simulink model "video_QPSK"  (R2024b)
settings: Solver=VariableStepAuto  StartTime=0.0  StopTime=10.0  RelTol=1e-3
values from neighbouring files (symbols this model uses):
  frame_rate = video.FrameRate    [vid.m]
undefined symbols (not defined in the file or in its folder): doppler, j
libraries: dspxfrm3 x3, commchan3 x2, commdigbbndpm3 x2, commsink2 x1, commeq3 x1
settings Model: Creator=戴文滔  LastModifiedBy=smz92

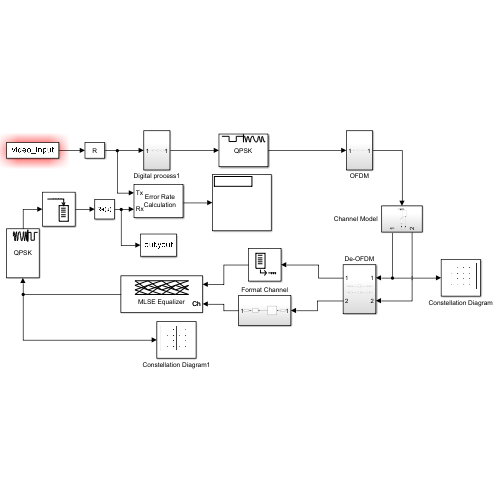
[thumbnail: Simulink's stored preview of the top-level diagram]
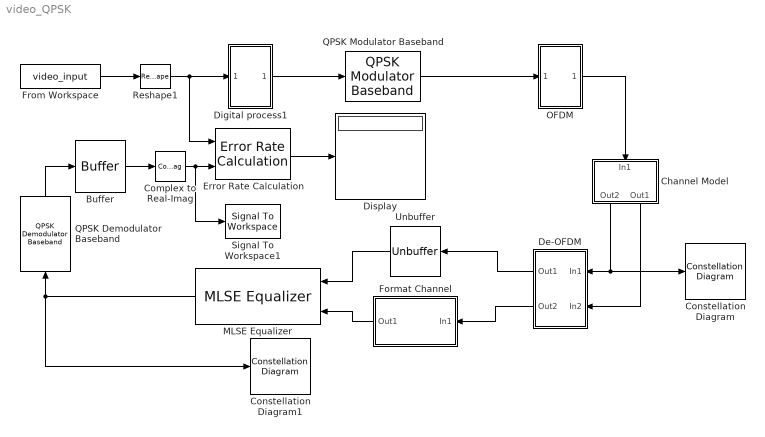
== system video_QPSK ==
  Buffer : Buffer  N=1  OutputFrames=off
  Channel Model : Subsystem
  Complex to Real-Imag : ComplexToRealImag  Output=Real
  Constellation Diagram : ConstellationDiagram  WindowPosition=[0.000000,-7.000000,1706.000000,937.000000,]  ScopeFrameLocation=window  XLimits=[-1.76,1.76]  YLimits=[-1.38,1.38]  ColorFading=on  MeasurementInterval=All displays
  Constellation Diagram1 : ConstellationDiagram  WindowPosition=[906.000000,121.000000,600.000000,600.000000,]  ScopeFrameLocation=window  XLimits=[-1.47,1.47]  YLimits=[-1.38,1.38]
  De-OFDM : Subsystem
  Digital process1 : Subsystem
  Display : Display
  Error Rate Calculation : commsink2/Error Rate Calculation  N=0  st_delay=0  cp_mode=Entire frame  subframe=[]  PMode=Port  WsName=ErrorVec  RsMode2=off  stop=off  numErr=100  maxBits=1e6
  Format Channel : Subsystem
  From Workspace : FromWorkspace  VariableName=video_input  SampleTime=1/frame_rate
  MLSE Equalizer : commeq3/MLSE Equalizer  specchan=Input port  chancoeff=[1 0.7 0.5 0.3]'  constpts=[1+j -1+j -1-j 1-j]  tbdepth=10  opmode=Continuous with reset option  enpreamble=off  preamble=[0 3 2 1]  enpostamble=off  postamble=[0 2 3 1]  numsamp=1  reset=off
  OFDM : Subsystem
  QPSK Demodulator Baseband : commdigbbndpm3/QPSK Demodulator Baseband  OutType=Integer  DecType=Hard decision  VarSource=Dialog  Variance=1  Dec=Gray  Ph=pi/4  outDtype1=Inherit via internal rule  outDtype2=Inherit via internal rule  derotateFactorWordLen=16  derotateFactorDataTypeStr=Inherit: Same word length as input  derotateFactorLastDataTypeStr=Inherit: Same word length as input
  QPSK Modulator Baseband : commdigbbndpm3/QPSK Modulator Baseband  InType=Integer  Enc=Gray  Ph=pi/4  outDtype=double  outWordLen=16  outUDDataType=sfix(16)  outFracLenMode=Best precision  outFracLen=15  outDataTypeStr=double  outLastDataTypeStr=double
  Reshape1 : Reshape  OutputDimensionality=Customize  OutputDimensions=[4096,1]
  Signal To Workspace1 : SignalToWorkspace  VariableName=yout
      settings: CopyFcn=dspblkcopystw(gcbh);
  Unbuffer : Unbuffer
  wires:
  Channel Model/2(Out1) -> De-OFDM/2(In2)
  MLSE Equalizer/1 -> QPSK Demodulator Baseband/1, Constellation Diagram1/1
  QPSK Demodulator Baseband/1 -> Buffer/1
  OFDM/1(Out1) -> Channel Model/1(In1)
  Format Channel/1(Out1) -> MLSE Equalizer/2
  De-OFDM/2(Out2) -> Format Channel/1(In1)
  Error Rate Calculation/1 -> Display/1
  Buffer/1 -> Complex to Real-Imag/1
  Unbuffer/1 -> MLSE Equalizer/1
  De-OFDM/1(Out1) -> Unbuffer/1
  QPSK Modulator Baseband/1 -> OFDM/1(In1)
  Channel Model/1(Out2) -> Constellation Diagram/1, De-OFDM/1(In1)
  Digital process1/1(Out1) -> QPSK Modulator Baseband/1
  From Workspace/1 -> Reshape1/1
  Reshape1/1 -> Error Rate Calculation/1, Digital process1/1(In1)
  Complex to Real-Imag/1 -> Signal To Workspace1/1, Error Rate Calculation/2

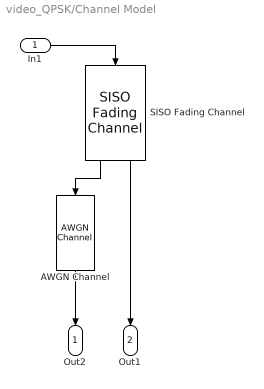
== system video_QPSK/Channel Model ==
  In1 : Inport
  AWGN Channel : commchan3/AWGN Channel  LegacyMode=off  NoiseMethod="Signal to noise ratio  (Eb/No)"  noiseMode="Signal to noise ratio  (SNR)"  EbNo=10  EsNo=10  SNR=10  BitsPerSymbol=1  SignalPower=1  SamplesPerSymbol=1  SymbolPeriod=1  VarianceSource=Parameter  Variance=1  RandomStream=Global stream  Seed=67  SimulateUsing=Interpreted execution
  SISO Fading Channel : commchan3/SISO Fading Channel  InheritSampleRate=on  SampleRate=1  PathDelays=0  AveragePathGains=0  NormalizePathGains=on  FadingDistribution=Rayleigh  KFactor=3  DirectPathDopplerShift=0  DirectPathInitialPhase=0  MaximumDopplerShift=0.001  DopplerSpectrum=doppler('Jakes')  RandomStream=mt19937ar with seed  Seed=73  PathGainsOutputPort=on  ChannelFilterDelayOutputPort=off  SimulateUsing=Interpreted execution  Visualization=Off  PathsForDopplerDisplay=1  SamplesToDisplay=25%
  Out2 : Outport
  Out1 : Outport  Port=2
  wires:
  In1/1 -> SISO Fading Channel/1
  AWGN Channel/1 -> Out2/1
  SISO Fading Channel/1 -> AWGN Channel/1
  SISO Fading Channel/2 -> Out1/1

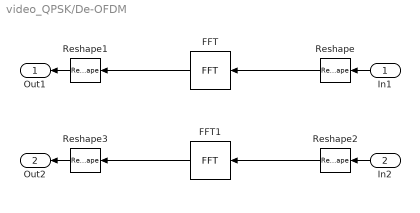
== system video_QPSK/De-OFDM ==
  In1 : Inport
  In2 : Inport  Port=2
  FFT : dspxfrm3/FFT  FFTImplementation=Auto  CompMethod=Table lookup  TableOpt=NEW  TableOptActive=Speed  BitRevOrder=off  Normalize=off  InheritFFTLength=on  FFTLength=64  WrapInput=on  roundingMode=Ceiling  overflowMode=off  firstCoeffDataTypeStr=Inherit: Same word length as input  firstCoeffLastDataTypeStr=Inherit: Same word length as input  outputMin=[]  outputMax=[]
  FFT1 : dspxfrm3/FFT  FFTImplementation=Auto  CompMethod=Table lookup  TableOpt=NEW  TableOptActive=Speed  BitRevOrder=off  Normalize=off  InheritFFTLength=on  FFTLength=64  WrapInput=on  roundingMode=Ceiling  overflowMode=off  firstCoeffDataTypeStr=Inherit: Same word length as input  firstCoeffLastDataTypeStr=Inherit: Same word length as input  outputMin=[]  outputMax=[]
  Reshape{,1..3} (4 alike) : Reshape
  Out1 : Outport
  Out2 : Outport  Port=2
  wires:
  FFT/1 -> Reshape1/1
  Reshape/1 -> FFT/1
  In1/1 -> Reshape/1
  Reshape1/1 -> Out1/1
  Reshape3/1 -> Out2/1
  In2/1 -> Reshape2/1
  Reshape2/1 -> FFT1/1
  FFT1/1 -> Reshape3/1

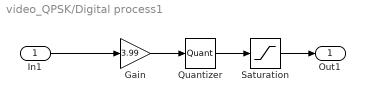
== system video_QPSK/Digital process1 ==
  In1 : Inport
  Gain : Gain  Gain=3.99
  Quantizer : Quantizer  QuantizationInterval=1
  Saturation : Saturate  UpperLimit=3  LowerLimit=0
  Out1 : Outport
  wires:
  Gain/1 -> Quantizer/1
  Quantizer/1 -> Saturation/1
  Saturation/1 -> Out1/1
  In1/1 -> Gain/1

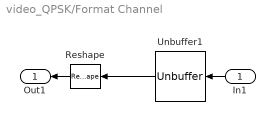
== system video_QPSK/Format Channel ==
  In1 : Inport
  Reshape : Reshape
  Unbuffer1 : Unbuffer
  Out1 : Outport
  wires:
  Reshape/1 -> Out1/1
  Unbuffer1/1 -> Reshape/1
  In1/1 -> Unbuffer1/1

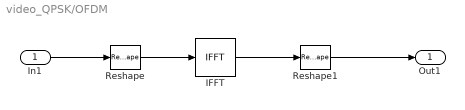
== system video_QPSK/OFDM ==
  In1 : Inport
  IFFT : dspxfrm3/IFFT  FFTImplementation=Auto  CompMethod=Table lookup  TableOpt=NEW  TableOptActive=Speed  BitRevOrder=off  cs_in=off  Normalize=on  InheritFFTLength=on  FFTLength=64  WrapInput=on  mode=Real  outSamplingMode=Sample based  roundingMode=Ceiling  overflowMode=off  firstCoeffDataTypeStr=Inherit: Same word length as input  firstCoeffLastDataTypeStr=Inherit: Same word length as input  outputMin=[]  outputMax=[]
  Reshape : Reshape
  Reshape1 : Reshape  OutputDimensions=[2,1]
  Out1 : Outport
  wires:
  In1/1 -> Reshape/1
  Reshape1/1 -> Out1/1
  Reshape/1 -> IFFT/1
  IFFT/1 -> Reshape1/1
